simulink model "reproiectare_RST"  (R2020a)
settings: Solver=VariableStepAuto  StartTime=0.0  StopTime=100  RelTol=1e-3
settings Model: Creator=user  LastModifiedBy=user

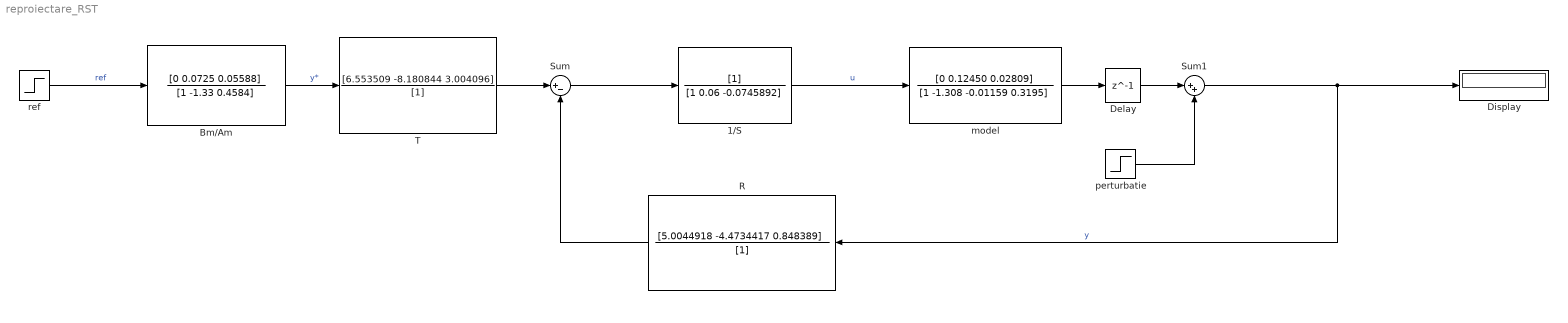
== system reproiectare_RST ==
  1/S : DiscreteFilter  Denominator=[1 0.06 -0.0745892]  SampleTime=0.6
  Bm/Am : DiscreteFilter  Numerator=[0 0.0725 0.05588]  Denominator=[1 -1.33 0.4584]  SampleTime=0.6
  Delay : Delay  DelayLength=1  SampleTime=0.6
  Display : Display
  R : DiscreteFilter  Numerator=[5.0044918 -4.4734417 0.848389]  Denominator=[1]  SampleTime=0.6
  Sum : Sum  Inputs=|+-
  Sum1 : Sum  Inputs=|++
  T : DiscreteFilter  Numerator=[6.553509 -8.180844 3.004096]  Denominator=[1]  SampleTime=0.6
  model : DiscreteFilter  Numerator=[0 0.12450 0.02809]  Denominator=[1 -1.308 -0.01159 0.3195]  SampleTime=0.6
  perturbatie : Step  Time=50  After=0.25  SampleTime=0.6
  ref : Step  SampleTime=0.6
  wires:
  R/1 -> Sum/2
  T/1 -> Sum/1
  model/1 -> Delay/1
  Sum/1 -> 1/S/1
  perturbatie/1 -> Sum1/2
  1/S/1 -> model/1  "u"
  ref/1 -> Bm/Am/1  "ref"
  Bm/Am/1 -> T/1  "y*"
  Sum1/1 -> Display/1, R/1  "y"
  Delay/1 -> Sum1/1
